simulink model "Lab14PIDs_2018a"  (R2018a)
settings: Solver=ode45  StartTime=0.0  StopTime=150  RelTol=1e-3  EnableMultiTasking=on
values from neighbouring files (symbols this model uses):
  A = [0 1 0 0 0 0; -Mg/I1 -B1psi/I1 0 0 b1/I1 0; 0 0 0 1 0 0; 0 0 0 -B1fi/I2 -kc*1.75*b1/I2 b2/I2; 0 0 0 0 -T10/T11 0; 0 0 0 0 0 -T20/T21]    [Lab14PID.m]    (also in linearizacao_planta.m = subs(jacobian(system,v),[x1 x2 x3 x4 x5 x6],[0 0 0 0 0 0]); trabalho_final_Simulacao.m = double(A))
  B = [0 0; 0 0; 0 0; 0 0; k1/T11 0; 0 k2/T21]    [Lab14PID.m]    (also in linearizacao_planta.m = subs(jacobian(system,v),[x1 x2 x3 x4 x5 x6],[0 0 0 0 0 0]); trabalho_final_Simulacao.m = double(B))
  C = [1 0 0 0 0 0; 0 0 1 0 0 0]    [Lab14PID.m]    (also in linearizacao_planta.m)
  D = [ 0 0; 0 0]    [Lab14PID.m]    (also in linearizacao_planta.m = 0)
  Ts = 0.1    [Lab14PID.m]
settings Model: Creator=morai
settings DataIOCC: LimitDataPoints=on
settings OptimizationCC: LifeSpan=inf
settings DebuggingCC: AllowSymbolicDim=off  SFUnexpectedBacktrackingDiag=warning  SFNoUnconditionalDefaultTransitionDiag=warning  SFExecutionAtInitializationDiag=none
settings ModelReferenceCC: PropagateSignalLabelsOutOfModel=off
settings CodeAppCC: StateflowObjectComments=on
settings GRTTargetCC: TargetLangStandard=C89/C90 (ANSI)
settings ConfigComp: CovMetricSettings=dw  CovSaveCumulativeToWorkspaceVar=on  CovSaveSingleToWorkspaceVar=on  CovExternalEMLEnable=off

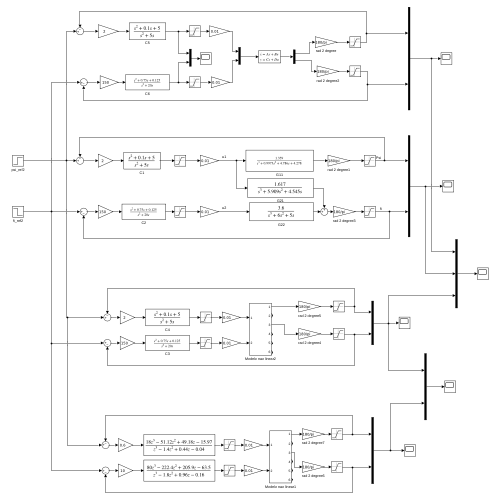
[thumbnail: Simulink's stored preview of the top-level diagram]
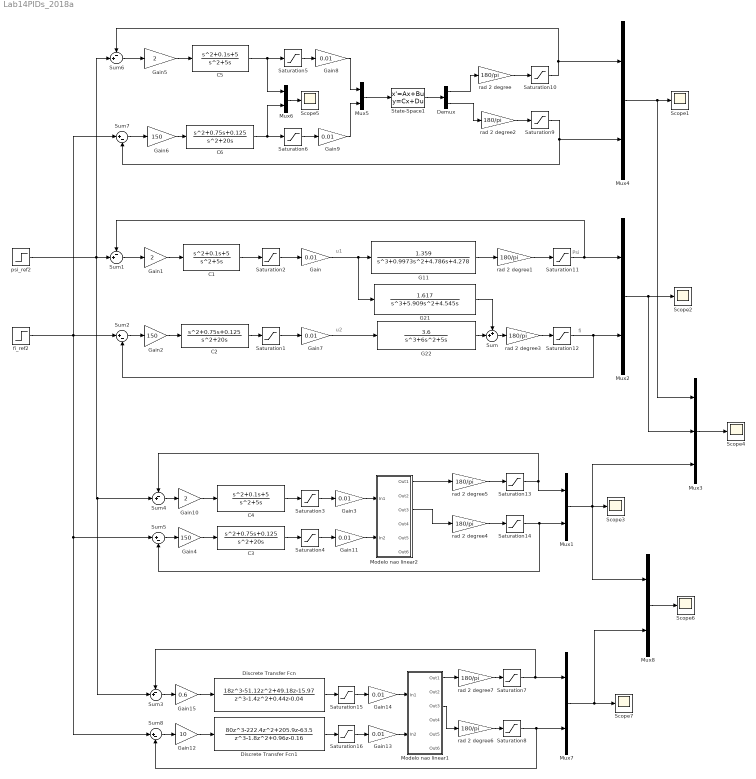
== system Lab14PIDs_2018a ==
  note: fi
  note: Psi
  note: u2
  note: u1
  C1 : TransferFcn  Numerator=[1 0.1 5]  Denominator=[1 5 0]
  C2 : TransferFcn  Numerator=[1 0.75 0.125]  Denominator=[1 20 0]
  C3 : TransferFcn  Numerator=[1 0.75 0.125]  Denominator=[1 20 0]
  C4 : TransferFcn  Numerator=[1 0.1 5]  Denominator=[1 5 0]
  C5 : TransferFcn  Numerator=[1 0.1 5]  Denominator=[1 5 0]
  C6 : TransferFcn  Numerator=[1 0.75 0.125]  Denominator=[1 20 0]
  Demux : Demux  Outputs=2
  Discrete Transfer Fcn : DiscreteTransferFcn  Numerator=[18 -51.12 49.18 -15.97]  Denominator=[1 -1.4 0.44 -0.04]  SampleTime=Ts
  Discrete Transfer Fcn1 : DiscreteTransferFcn  Numerator=[80 -222.4 205.9 -63.5]  Denominator=[1 -1.8 0.96 -0.16]  SampleTime=Ts
  G11 : TransferFcn  Numerator=[1.359]  Denominator=[1 0.9973 4.786 4.278]
  G21 : TransferFcn  Numerator=[1.617]  Denominator=[1 5.909 4.545 0]
  G22 : TransferFcn  Numerator=[3.6]  Denominator=[1 6 5 0]
  Gain{,3,7..9,11,13..14} (8 alike) : Gain  Gain=0.01
  Gain1 : Gain  Gain=2
  Gain10 : Gain  Gain=2
  Gain12 : Gain  Gain=10
  Gain15 : Gain  Gain=0.6
  Gain2 : Gain  Gain=150
  Gain4 : Gain  Gain=150
  Gain5 : Gain  Gain=2
  Gain6 : Gain  Gain=150
  Modelo nao linear1 : Subsystem
  Modelo nao linear2 : Subsystem
  Mux{1..2,4..8} (7 alike) : Mux  Inputs=2
  Mux3 : Mux  Inputs=3
  Saturation{1..6,15..16} (8 alike) : Saturate  UpperLimit=255  LowerLimit=-255
  Saturation{7,10..11,13} (4 alike) : Saturate  UpperLimit=80  LowerLimit=-80
  Saturation{8..9,12,14} (4 alike) : Saturate  UpperLimit=180  LowerLimit=-180
  Scope{1..7} (7 alike) : Scope
  State-Space1 : StateSpace  A=A  B=B  C=C  D=D  InitialCondition=0
  Sum : Sum  Inputs=++|
  Sum{1,3..4,6} (4 alike) : Sum  Inputs=-+|
  Sum{2,5,7..8} (4 alike) : Sum  Inputs=|+-
  fi_ref2 : Step  Time=70  Before=160  After=50  SampleTime=0
  psi_ref2 : Step  Time=40  Before=-32  After=0  SampleTime=0
  rad 2 degree{,1..7} (8 alike) : Gain  Gain=180/pi
  wires:
  C1/1 -> Saturation2/1
  G21/1 -> Sum/1
  G22/1 -> Sum/2
  C2/1 -> Saturation1/1
  Gain2/1 -> C2/1
  Sum2/1 -> Gain2/1
  Gain1/1 -> C1/1
  Sum1/1 -> Gain1/1
  psi_ref2/1 -> Sum3/2, Sum4/2, Sum6/2, Sum1/2
  Mux3/1 -> Scope4/1
  Mux2/1 -> Scope2/1, Mux3/2
  fi_ref2/1 -> Sum8/1, Sum5/1, Sum7/1, Sum2/1
  Gain6/1 -> C6/1
  Sum7/1 -> Gain6/1
  Gain5/1 -> C5/1
  Sum6/1 -> Gain5/1
  Mux5/1 -> State-Space1/1
  State-Space1/1 -> Demux/1
  Mux4/1 -> Mux3/1, Scope1/1
  Demux/1 -> rad 2 degree/1
  rad 2 degree/1 -> Saturation10/1
  Demux/2 -> rad 2 degree2/1
  rad 2 degree2/1 -> Saturation9/1
  Mux6/1 -> Scope5/1
  G11/1 -> rad 2 degree1/1
  rad 2 degree1/1 -> Saturation11/1
  Sum/1 -> rad 2 degree3/1
  rad 2 degree3/1 -> Saturation12/1
  Saturation2/1 -> Gain/1
  Gain/1 -> G21/1, G11/1
  Saturation1/1 -> Gain7/1
  Gain7/1 -> G22/1
  C5/1 -> Saturation5/1, Mux6/1
  Saturation5/1 -> Gain8/1
  Gain8/1 -> Mux5/1
  C6/1 -> Saturation6/1, Mux6/2
  Saturation6/1 -> Gain9/1
  Gain9/1 -> Mux5/2
  Saturation3/1 -> Gain3/1
  Gain3/1 -> Modelo nao linear2/1(In1)
  Saturation4/1 -> Gain11/1
  Gain11/1 -> Modelo nao linear2/2(In2)
  rad 2 degree4/1 -> Saturation14/1
  rad 2 degree5/1 -> Saturation13/1
  Mux8/1 -> Scope6/1
  Mux1/1 -> Mux8/1, Mux3/3, Scope3/1
  Gain4/1 -> C3/1
  Sum5/1 -> Gain4/1
  C3/1 -> Saturation4/1
  C4/1 -> Saturation3/1
  Sum4/1 -> Gain10/1
  Gain10/1 -> C4/1
  Saturation10/1 -> Mux4/1, Sum6/1
  Saturation9/1 -> Sum7/2, Mux4/2
  Saturation11/1 -> Mux2/1, Sum1/1
  Saturation12/1 -> Sum2/2, Mux2/2
  Saturation13/1 -> Mux1/1, Sum4/1
  Saturation14/1 -> Sum5/2, Mux1/2
  Discrete Transfer Fcn1/1 -> Saturation16/1
  Saturation8/1 -> Sum8/2, Mux7/2
  Modelo nao linear1/1(Out1) -> rad 2 degree7/1
  Saturation16/1 -> Gain13/1
  Modelo nao linear1/3(Out3) -> rad 2 degree6/1
  Saturation15/1 -> Gain14/1
  Discrete Transfer Fcn/1 -> Saturation15/1
  rad 2 degree6/1 -> Saturation8/1
  Gain13/1 -> Modelo nao linear1/2(In2)
  Saturation7/1 -> Mux7/1, Sum3/1
  Gain14/1 -> Modelo nao linear1/1(In1)
  rad 2 degree7/1 -> Saturation7/1
  Mux7/1 -> Mux8/2, Scope7/1
  Sum8/1 -> Gain12/1
  Sum3/1 -> Gain15/1
  Gain12/1 -> Discrete Transfer Fcn1/1
  Gain15/1 -> Discrete Transfer Fcn/1
  Modelo nao linear2/3(Out3) -> rad 2 degree4/1
  Modelo nao linear2/1(Out1) -> rad 2 degree5/1

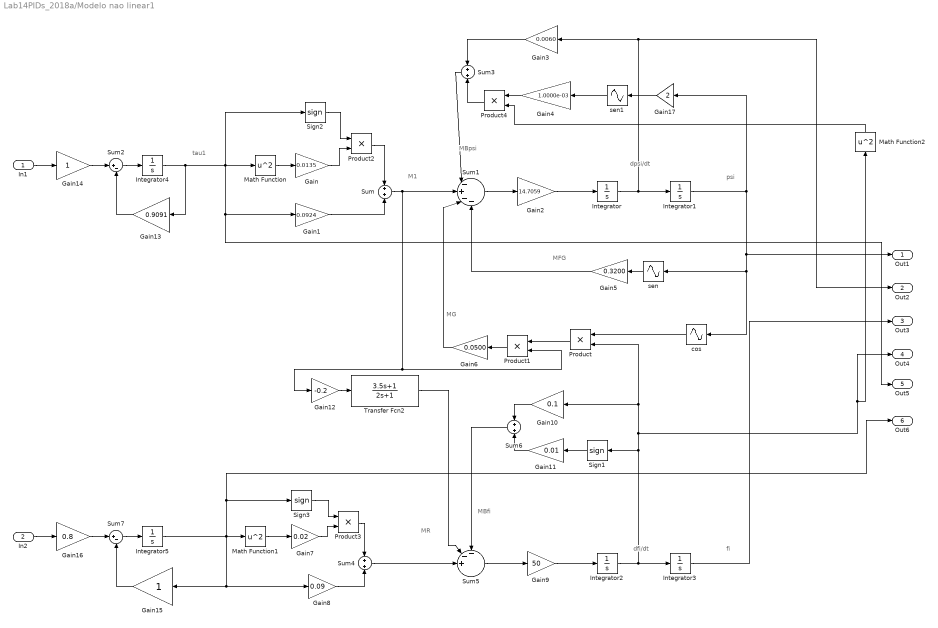
== system Lab14PIDs_2018a/Modelo nao linear1 ==
  note: MBfi
  note: MR
  note: psi
  note: MFG
  note: tau1
  note: M1
  note: MG
  note: MBpsi
  note: fi
  note: dfi/dt
  note: dpsi/dt
  In1 : Inport
  In2 : Inport  Port=2
  Gain : Gain  Gain=0.0135
  Gain1 : Gain  Gain=0.0924
  Gain10 : Gain  Gain=0.1
  Gain11 : Gain  Gain=0.01
  Gain12 : Gain  Gain=-0.2
  Gain13 : Gain  Gain=0.9091
  Gain14 : Gain
  Gain15 : Gain
  Gain16 : Gain  Gain=0.8
  Gain17 : Gain  Gain=2
  Gain2 : Gain  Gain=14.7059
  Gain3 : Gain  Gain=0.0060
  Gain4 : Gain  Gain=1.0000e-03
  Gain5 : Gain  Gain=0.3200
  Gain6 : Gain  Gain=0.0500
  Gain7 : Gain  Gain=0.02
  Gain8 : Gain  Gain=0.09
  Gain9 : Gain  Gain=50
  Integrator{,1..5} (6 alike) : Integrator
  Math Function : Math  Operator=square  SaturateOnIntegerOverflow=on
  Math Function1 : Math  Operator=square  SaturateOnIntegerOverflow=on
  Math Function2 : Math  Operator=square  SaturateOnIntegerOverflow=on
  Product{,1..4} (5 alike) : Product
  Sign1 : Signum  ZeroCross=off
  Sign2 : Signum  ZeroCross=off
  Sign3 : Signum  ZeroCross=off
  Sum{,3..4,6} (4 alike) : Sum
  Sum1 : Sum  Inputs=|-+--
  Sum2 : Sum  Inputs=|+-
  Sum5 : Sum  Inputs=--+||
  Sum7 : Sum  Inputs=|+-
  Transfer Fcn2 : TransferFcn  Numerator=[3.5 1]  Denominator=[2 1]
  cos : Sin  TimeSource=Use external signal  Phase=pi/2  SampleTime=0
  sen : Sin  TimeSource=Use external signal  SampleTime=0
  sen1 : Sin  TimeSource=Use external signal  SampleTime=0
  Out1 : Outport  VectorParamsAs1DForOutWhenUnconnected=off
  Out2 : Outport  Port=2  VectorParamsAs1DForOutWhenUnconnected=off
  Out3 : Outport  Port=3  VectorParamsAs1DForOutWhenUnconnected=off
  Out4 : Outport  Port=4  VectorParamsAs1DForOutWhenUnconnected=off
  Out5 : Outport  Port=5  VectorParamsAs1DForOutWhenUnconnected=off
  Out6 : Outport  Port=6  VectorParamsAs1DForOutWhenUnconnected=off
  wires:
  Gain14/1 -> Sum2/1
  Integrator5/1 -> Math Function1/1, Sign3/1, Out6/1, Gain8/1, Gain15/1
  Sum2/1 -> Integrator4/1
  Gain15/1 -> Sum7/2
  Gain13/1 -> Sum2/2
  In1/1 -> Gain14/1
  Gain16/1 -> Sum7/1
  Sum7/1 -> Integrator5/1
  Integrator4/1 -> Gain13/1, Sign2/1, Math Function/1, Out5/1, Gain1/1
  Math Function/1 -> Gain/1
  Gain1/1 -> Sum/2
  Sum1/1 -> Gain2/1
  Gain2/1 -> Integrator/1
  Gain3/1 -> Sum3/1
  Sum3/1 -> Sum1/1
  Sum/1 -> Product1/2, Gain12/1, Sum1/2
  Integrator1/1 -> cos/1, sen/1, Out1/1, Gain17/1
  sen/1 -> Gain5/1
  Gain5/1 -> Sum1/4
  cos/1 -> Product/1
  Integrator2/1 -> Product/2, Gain10/1, Out4/1, Math Function2/1, Sign1/1, Integrator3/1
  Product1/1 -> Gain6/1
  Gain6/1 -> Sum1/3
  Product/1 -> Product1/1
  Math Function1/1 -> Gain7/1
  Gain8/1 -> Sum4/2
  Sum5/1 -> Gain9/1
  Gain9/1 -> Integrator2/1
  Sign1/1 -> Gain11/1
  Gain10/1 -> Sum6/1
  Gain11/1 -> Sum6/2
  In2/1 -> Gain16/1
  Integrator3/1 -> Out3/1
  Sum4/1 -> Sum5/3
  Sum6/1 -> Sum5/1
  Transfer Fcn2/1 -> Sum5/2
  Gain12/1 -> Transfer Fcn2/1
  Sign2/1 -> Product2/1
  Gain/1 -> Product2/2
  Product2/1 -> Sum/1
  Gain7/1 -> Product3/2
  Sign3/1 -> Product3/1
  Product3/1 -> Sum4/1
  sen1/1 -> Gain4/1
  Gain17/1 -> sen1/1
  Integrator/1 -> Out2/1, Gain3/1, Integrator1/1
  Gain4/1 -> Product4/1
  Product4/1 -> Sum3/2
  Math Function2/1 -> Product4/2

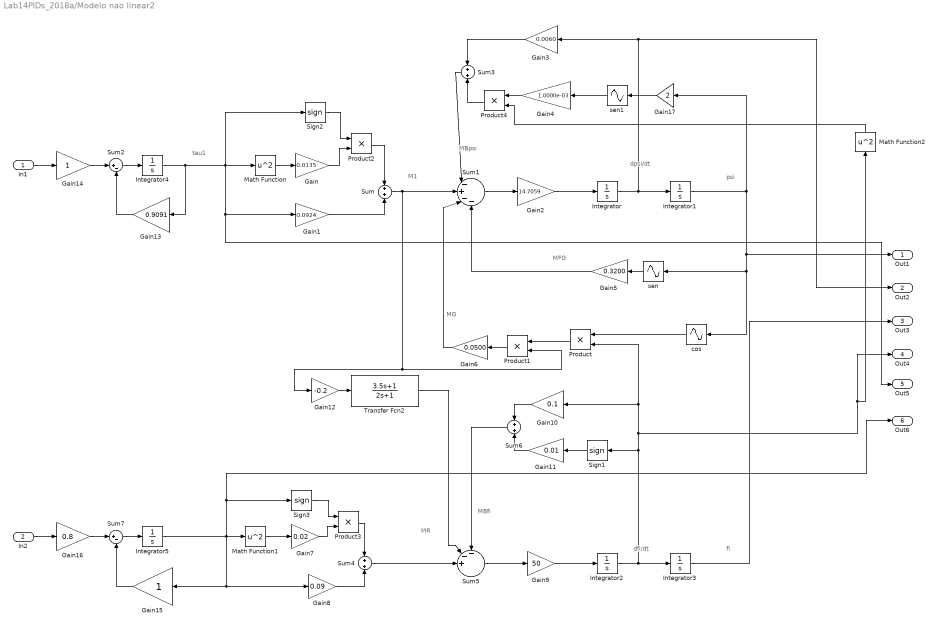
== system Lab14PIDs_2018a/Modelo nao linear2 ==
  note: MBfi
  note: MR
  note: psi
  note: MFG
  note: tau1
  note: M1
  note: MG
  note: MBpsi
  note: fi
  note: dfi/dt
  note: dpsi/dt
  In1 : Inport
  In2 : Inport  Port=2
  Gain : Gain  Gain=0.0135
  Gain1 : Gain  Gain=0.0924
  Gain10 : Gain  Gain=0.1
  Gain11 : Gain  Gain=0.01
  Gain12 : Gain  Gain=-0.2
  Gain13 : Gain  Gain=0.9091
  Gain14 : Gain
  Gain15 : Gain
  Gain16 : Gain  Gain=0.8
  Gain17 : Gain  Gain=2
  Gain2 : Gain  Gain=14.7059
  Gain3 : Gain  Gain=0.0060
  Gain4 : Gain  Gain=1.0000e-03
  Gain5 : Gain  Gain=0.3200
  Gain6 : Gain  Gain=0.0500
  Gain7 : Gain  Gain=0.02
  Gain8 : Gain  Gain=0.09
  Gain9 : Gain  Gain=50
  Integrator{,1..5} (6 alike) : Integrator
  Math Function : Math  Operator=square  SaturateOnIntegerOverflow=on
  Math Function1 : Math  Operator=square  SaturateOnIntegerOverflow=on
  Math Function2 : Math  Operator=square  SaturateOnIntegerOverflow=on
  Product{,1..4} (5 alike) : Product
  Sign1 : Signum  ZeroCross=off
  Sign2 : Signum  ZeroCross=off
  Sign3 : Signum  ZeroCross=off
  Sum{,3..4,6} (4 alike) : Sum
  Sum1 : Sum  Inputs=|-+--
  Sum2 : Sum  Inputs=|+-
  Sum5 : Sum  Inputs=--+||
  Sum7 : Sum  Inputs=|+-
  Transfer Fcn2 : TransferFcn  Numerator=[3.5 1]  Denominator=[2 1]
  cos : Sin  TimeSource=Use external signal  Phase=pi/2  SampleTime=0
  sen : Sin  TimeSource=Use external signal  SampleTime=0
  sen1 : Sin  TimeSource=Use external signal  SampleTime=0
  Out1 : Outport  VectorParamsAs1DForOutWhenUnconnected=off
  Out2 : Outport  Port=2  VectorParamsAs1DForOutWhenUnconnected=off
  Out3 : Outport  Port=3  VectorParamsAs1DForOutWhenUnconnected=off
  Out4 : Outport  Port=4  VectorParamsAs1DForOutWhenUnconnected=off
  Out5 : Outport  Port=5  VectorParamsAs1DForOutWhenUnconnected=off
  Out6 : Outport  Port=6  VectorParamsAs1DForOutWhenUnconnected=off
  wires:
  Gain14/1 -> Sum2/1
  Integrator5/1 -> Math Function1/1, Sign3/1, Out6/1, Gain8/1, Gain15/1
  Sum2/1 -> Integrator4/1
  Gain15/1 -> Sum7/2
  Gain13/1 -> Sum2/2
  In1/1 -> Gain14/1
  Gain16/1 -> Sum7/1
  Sum7/1 -> Integrator5/1
  Integrator4/1 -> Gain13/1, Sign2/1, Math Function/1, Out5/1, Gain1/1
  Math Function/1 -> Gain/1
  Gain1/1 -> Sum/2
  Sum1/1 -> Gain2/1
  Gain2/1 -> Integrator/1
  Gain3/1 -> Sum3/1
  Sum3/1 -> Sum1/1
  Sum/1 -> Product1/2, Gain12/1, Sum1/2
  Integrator1/1 -> cos/1, sen/1, Out1/1, Gain17/1
  sen/1 -> Gain5/1
  Gain5/1 -> Sum1/4
  cos/1 -> Product/1
  Integrator2/1 -> Product/2, Gain10/1, Out4/1, Math Function2/1, Sign1/1, Integrator3/1
  Product1/1 -> Gain6/1
  Gain6/1 -> Sum1/3
  Product/1 -> Product1/1
  Math Function1/1 -> Gain7/1
  Gain8/1 -> Sum4/2
  Sum5/1 -> Gain9/1
  Gain9/1 -> Integrator2/1
  Sign1/1 -> Gain11/1
  Gain10/1 -> Sum6/1
  Gain11/1 -> Sum6/2
  In2/1 -> Gain16/1
  Integrator3/1 -> Out3/1
  Sum4/1 -> Sum5/3
  Sum6/1 -> Sum5/1
  Transfer Fcn2/1 -> Sum5/2
  Gain12/1 -> Transfer Fcn2/1
  Sign2/1 -> Product2/1
  Gain/1 -> Product2/2
  Product2/1 -> Sum/1
  Gain7/1 -> Product3/2
  Sign3/1 -> Product3/1
  Product3/1 -> Sum4/1
  sen1/1 -> Gain4/1
  Gain17/1 -> sen1/1
  Integrator/1 -> Out2/1, Gain3/1, Integrator1/1
  Gain4/1 -> Product4/1
  Product4/1 -> Sum3/2
  Math Function2/1 -> Product4/2
